simulink model "MCU_ExternalModeDataLog_dsPIC33AK128MC106"  (R2024a)
settings: Solver=FixedStepDiscrete  StartTime=0.0  StopTime=inf  FixedStep=50e-6  RelTol=1e-3  EnableMultiTasking=on
undefined symbols (not defined in the file or in its folder): A0, A4, ADC, B0, C10, C11, C6, C7, C8, control, D11, D12, DiscIntNeverNeededParam, inverter, Max, MaxPer, motor, ms, NumBits1, NumBits2, P1, P17, P20, P39, P40, P41, P43, P44, P60, P61, Pin, PosRange1, PosRange2, PWM1_Trg1, Resol, s, Slope1, Slope2, us
libraries: simulink x34, MCHP_Blockset x18
(part 1 of 5)
settings Model: SimulationMode=external  ExtModeEnableFloating=off  ExtModeTrigDuration=20  Creator=rdelpoux  LastModifiedBy=rdelpoux
settings SolverCC: AlgebraicLoopSolver=TrustRegion
settings OptimizationCC: DefaultParameterBehavior=Inlined  DefaultUnderspecifiedDataType=single  EnhancedBackFolding=on  BooleansAsBitfields=on  PassReuseOutputArgsAs=Individual arguments  ZeroExternalMemoryAtStartup=off  ZeroInternalMemoryAtStartup=off  OptimizeBlockOrder=speed  DifferentSizesBufferReuse=on  EfficientTunableParamExpr=on
settings DebuggingCC: MultiTaskDSMMsg=none  MultiTaskCondExecSysMsg=none  MultiTaskRateTransMsg=warning  ParameterTunabilityLossMsg=error  ArithmeticOperatorsInVariantConditions=warning
settings HardwareCC: ProdBitPerPointer=32  ProdBitPerSizeT=32  ProdBitPerPtrDiffT=32  ProdLargestAtomicInteger=Long  ProdWordSize=32  ProdLongLongMode=on  ProdHWDeviceType=Generic->Custom
settings ModelReferenceCC: ModelReferenceNumInstancesAllowed=Single
settings SFSimCC: MATLABDynamicMemAlloc=off  CustomCodeUndefinedFunction=UseInterfaceOnly
settings RTWCC: Description=Microchip Embedded Target dsPIC33A (real-time)  SystemTargetFile=MCHP_dsPIC33A_stf.tlc  TLCOptions=-aExtModeXCPClassicInterface=0  TemplateMakefile=MCHP_dsPIC33A.tmf  GPUComputeCapability=3.5
settings CodeAppCC: ForceParamTrailComments=on  IgnoreCustomStorageClasses=off  MaxIdLength=255  OperatorAnnotations=on  SimulinkDataObjDesc=on  SFDataObjDesc=on  InsertBlockDesc=on
settings STFCustomTargetCC: TargetLibSuffix=_lib.a  MultiwordLength=256  CombineOutputUpdateFcns=on  CombineSignalStateStructs=on  ERTCustomFileBanners=on  SupportContinuousTime=off  RemoveResetFunc=on  MATLABClassNameForMDSCustomization=Simulink.SoftwareTarget.ERTCustomization  GRTInterface=off  UseToolchainInfoCompliant=off  SystemTargetFile=MCHP_dsPIC33A_stf.tlc
settings ERTTargetCC: TargetLibSuffix=_lib.a  TargetLangStandard=C99 (ISO)  ParMdlRefBuildCompliant=off  CompOptLevelCompliant=off  ConcurrentExecutionCompliant=off  CombineSignalStateStructs=on  SupportNonInlinedSFcns=on  ModelStepFunctionPrototypeControlCompliant=off  CPPClassGenCompliant=off  UseToolchainInfoCompliant=off  ExtMode=on  ExtModeTransport=1  ExtModeStaticAlloc=on  ExtModeStaticAllocSize=2048  ExtModeMexFile=ext_xcp  ExtModeMexArgs=1 '/dev/ttyACM1' 460800 './MCU_LuenbergerObserver_dsPIC33AK128MC106.X/MCU_LuenbergerObserver_dsPIC33AK128MC106.elf'  ExtModeIntrfLevel=Level2 - Open  InlinedParameterPlacement=NonHierarchical  ERTSrcFileBannerTemplate=MCHP_dsPIC_code_template.cgt  ERTHdrFileBannerTemplate=MCHP_dsPIC_code_template.cgt  ERTDataSrcFileTemplate=MCHP_dsPIC_code_template.cgt  ERTDataHdrFileTemplate=MCHP_dsPIC_code_template.cgt  ERTCustomFileTemplate=MCHP_main.tlc  MaxLineWidth=110

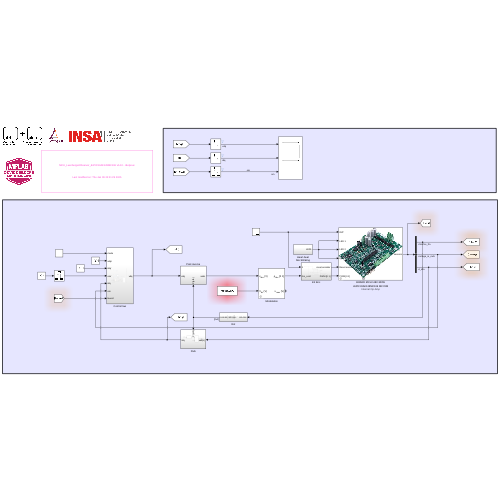
[thumbnail: Simulink's stored preview of the top-level diagram]
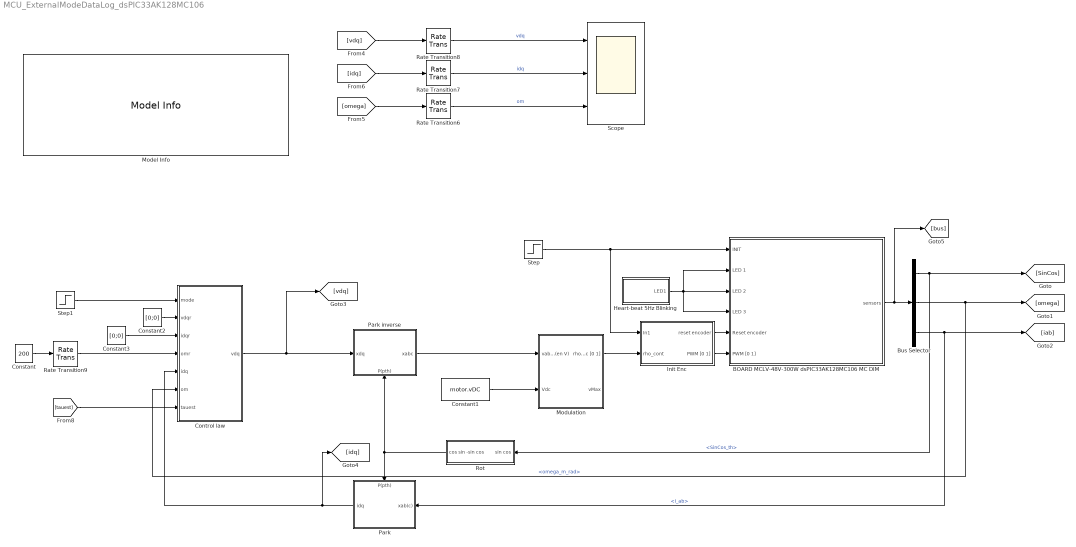
== system MCU_ExternalModeDataLog_dsPIC33AK128MC106 ==
  BOARD MCLV-48V-300W dsPIC33AK128MC106 MC DIM : Subsystem  mask(MCLV-48V-300W - dsPIC33AK128MC106 MC DIM){boardVariants=Internal Op-Amp, n=4, QEIResolution=4000, Switching_Frequency=20000, DeadTime=1e-6, QEI_Reset=on index signal, QEI_Offset_settings=0, QEIOffset=0.1885}
      mask prompts: boardVariants "Board Variants"; n "Motor Pole Pairs"; QEIResolution "Optical Encoder Resolution Per Mechanical Rotation (lines)"; Switching_Frequency "PWM Switching Frequency (Hz)"; DeadTime "Dead Time (s)"; QEI_Reset "Optical encoder reset"; QEI_Offset_settings "Optical encoder offset (mechanical in rad)"; QEIOffset "Optical encoder offset (mechanical in rad)"
      mask help:
      | Template for motor control board MCLV-48V-300W with the dsPIC33AK128MC106 Motor Control DIM.
      |
      | Block bus output provices:
      |   - Current phase ia & ib, DC bus and potentiometer position
      |   - Buttons (0 when pressed, 1 for Btn 3 unconnected)
      |   - QEI position and velocity
      |   - MCU load and overload
      |
      | Block inputs:
      |   - INIT signal average the current phase ia and ib to be removed
      |   - LEDs
      |   - Reset encoder allows to align the motor while reseting the encoder
      |   - PWM normalized duty cycle value
      |
      | Model 50us base rate (20kHz) is synchronized with ADC conversion which is synchronized with the 50us PWM periods
      mask init:
      | BlksQEI = find_system(gcb,'FollowLinks','on','LookUnderMasks','all','ReferenceBlock','MCHP_Blockset/QEI/QEI');
      | QEI_Reset = get_param(gcb,'QEI_Reset');
      | if numel(BlksQEI) >= 1
      |     switch QEI_Reset
      |         case 'on index signal'
      |             set_param(BlksQEI{1},'PIMOD_mode','RESET position on each INDEX event');
      |         case 'on logical input (software)'        
      |             set_param(BlksQEI{1},'PIMOD_mode','position is cyclique between user defined boundaries'); 
      |         case 'custom setting'
      |             % do nothing 
      |     end
      | end % if
      | 
      |     BlksOpAmp = find_system(gcb,'FollowLinks','on','IncludeCommented','on','LookUnderMasks','all','ReferenceBlock','MCHP_Blockset/Analog IO/Op-Amp');
      |     if numel(BlksOpAmp) >= 1
      |         boardVariants = get_param(gcb,'boardVariants');
      |         switch boardVariants
      |             case 'Internal Op-Amp'
      |                 set_param(BlksOpAmp{1},'Commented','off');
      |             case 'External Op-Amp'
      |                 set_param(BlksOpAmp{1},'Commented','on');
      |         end
      |     end % if
      settings: AttributesFormatString=%<boardVariants>
      mask Help: https://forum.microchip.com/s/sub-forums?&subForumId=a553l000000J2rNAAS&forumId=a553l000000J2pvAAC&subForumName=MATLAB&forumName=Development%20Tools&page=1&offset=0
      mask TypeOptions boardVariants: Internal Op-Amp | External Op-Amp
      mask TypeOptions QEI_Reset: on index signal | on logical input (software) | custom setting
      mask Callback QEI_Reset:
      | QEI_Reset = get_param(gcb,'QEI_Reset');
      | switch QEI_Reset
      |     case 'on index signal'
      |         QEIOffset = MCHP_Fun.Evalin('base','QEIOffset');
      |         set_param(gcb,'QEIOffset',num2str(QEIOffset));
      |         set_param(gcb,'MaskVisibilities',{'on';'on';'on';'on';'on';'on';'off';'on'});
      |     case 'on logical input (software)'
      |         set_param(gcb,'QEIOffset','0');
      |         set_param(gcb,'MaskVisibilities',{'on';'on';'on';'on';'on';'on';'off';'off'});
      |     case 'custom setting'
      |         set_param(gcb,'MaskVisibilities',{'on';'on';'on';'on';'on';'on';'off';'on'});
      |         % do nothing
      | end
      mask DialogControl boardParameters Prompt: Board
      mask DialogControl MotorParameters Prompt: Motor
      mask DialogControl n Tooltip: Number of pole pairs of the motor
      mask DialogControl QEIResolution Tooltip: encoder resolution per mechanical rotation
      mask DialogControl PWMParameters Prompt: PWM
      mask DialogControl QEIParameters Prompt: QEI
      mask DialogControl QEI_Reset Tooltip: enable encoder index signal if available. Otherwise align motor by applying a tension and set the rst input to 1
      mask DialogControl QEI_Offset_settings Tooltip: offset angle between encoder index and motor winding reference axis applied on theta_m and theta_e
      mask Display: image('MCHP_i_Board_MCLV_300W48V_reduced.jpg');
  Bus Selector : BusSelector  OutputSignals=optical coder.elec.SinCos_th,optical coder.mecc.omega_m_rad,ADC.I_ab
  Constant : Constant  Value=200
  Constant1 : Constant  Value=motor.vDC  OutDataTypeStr=single
  Constant2 : Constant  Value=[0;0]  OutDataTypeStr=single
  Constant3 : Constant  Value=[0;0]  OutDataTypeStr=single
  Control law : Subsystem
      settings: LibrarySourceBlock=insa_control_base/Control law
  Heart-beat 5Hz Blinking : Subsystem
  Init Enc : Subsystem
  Model Info : simulink/Model-Wide Utilities/Model Info  Frame=on  DisplayStringWithTags=|  HorizontalTextAlignment=Center  LeftAlignmentValue=0.5
      | %<ModelName> v%<ModelVersion> - %<Creator>
      | 
      | %<Description>
      | 
      | Last modified on: %<LastModificationDate>
  Modulation : Subsystem  mask{modulation=Space Vector, mod=0}
      mask init:
      | switch modulation
      |     case 'Sinusoidale'
      |         mod = 0;
      |     otherwise
      |         mod = 1;
      | end
      mask TypeOptions modulation: Sinusoidale | Space Vector
      mask DialogControl DescGroupVar Prompt: Modulation interssecticve
      mask DialogControl DescTextVar Prompt: Choose between sinus or space vector modulation
      mask Display:
      | port_label('output', 1, '\rho_{abc} [0 1]', 'texmode','on')
      | port_label('output', 2, 'v_{\rm max} (V)', 'texmode','on')
      | port_label('input', 1, 'v_{abc} (V)', 'texmode','on')
      | port_label('input', 2, 'V_{dc} (V)', 'texmode','on')
  Park : Subsystem
      settings: PortSchema="{\"entries\":[{\"content\":{\"sides\":[{\"content\":{\"connectorIds\":[\"In1\"]},\"type\":\"ConnectorPlacement.EquallySpacedRectSide\",\"uuid\":\"ebf2fcb8-f94c-4630-a735-fb74e68b604e\"},{\"content\":{\"connectorIds\":[\"Out1\"],\"side\":\"RIGHT\"},\"type\":\"ConnectorPlacement.EquallySpacedRectSide\",\"uuid\":\"fb89ad3f-9420-4065-992c-c6d77ce245e0\"},{\"content\":{\"connectorIds\":[\"In2\"],\"side\":\"TOP\"},\"type\":\"ConnectorPlacement.EquallySpacedRectSide\",\"uuid\":\"0249ceba-2241-48c9-87d4-d9d6f381f2d7\"}]},\"type\":\"ConnectorPlacement.EquallySpacedConnector\",\"uuid\":\"eecfd82d-5918-403e-a677-09fe1d8cc737\"}],\"packageUris\":[\"http://schema.mathworks.com/mf0/Connector/R2020b\"],\"version\":\"1.0\"}"
  Park inverse : Subsystem
      settings: PortSchema="{\"entries\":[{\"content\":{\"sides\":[{\"content\":{\"connectorIds\":[\"In1\"]},\"type\":\"ConnectorPlacement.EquallySpacedRectSide\",\"uuid\":\"4c11ef0a-1978-4a73-9b5c-4d5650fcee33\"},{\"content\":{\"connectorIds\":[\"Out1\"],\"side\":\"RIGHT\"},\"type\":\"ConnectorPlacement.EquallySpacedRectSide\",\"uuid\":\"28284572-70c7-45ef-9db5-4b5788e96454\"},{\"content\":{\"side\":\"TOP\"},\"type\":\"ConnectorPlacement.EquallySpacedRectSide\",\"uuid\":\"3a1fbce2-0868-491b-8e3a-2b3a7a0d615d\"},{\"content\":{\"connectorIds\":[\"In2\"],\"side\":\"BOTTOM\"},\"type\":\"ConnectorPlacement.EquallySpacedRectSide\",\"uuid\":\"e63426ef-821a-4774-a922-a3f70d9b2116\"}]},\"type\":\"ConnectorPlacement.EquallySpacedConnector\",\"uuid\":\"285593a5-8af6-47f2-83d9-d6ebce98de71\"}],\"packageUris\":[\"http://schema.mathworks.com/mf0/Connector/R2020b\"],\"version\":\"1.0\"}"
  Rate Transition6 : RateTransition  OutPortSampleTime=0.001
  Rate Transition7 : RateTransition  OutPortSampleTime=0.001
  Rate Transition8 : RateTransition  OutPortSampleTime=0.001
  Rate Transition9 : RateTransition  OutPortSampleTime=5e-5
  Rot : Subsystem
  Scope : Scope  NumInputPorts=3
  Step : Step  Before=1  After=0  SampleTime=5e-5
  Step1 : Step  After=3  SampleTime=5e-5
  wires:
  Bus Selector/2 -> [omega], Control law/6(om)  "<omega_m_rad>"
  BOARD MCLV-48V-300W dsPIC33AK128MC106 MC DIM/1(sensors) -> [bus], Bus Selector/1
  Bus Selector/1 -> Rot/1(sin cos), [SinCos]  "<SinCos_th>"
  Bus Selector/3 -> [iab], Park/1(xab(c))  "<I_ab>"
  Rot/1("cos sin -sin cos ") -> Park/2(P(pth)), Park inverse/2(P(pth))
  Constant1/1 -> Modulation/2(Vdc)
  Heart-beat 5Hz Blinking/1(LED1) -> BOARD MCLV-48V-300W dsPIC33AK128MC106 MC DIM/4(LED 3), BOARD MCLV-48V-300W dsPIC33AK128MC106 MC DIM/2(LED 1), BOARD MCLV-48V-300W dsPIC33AK128MC106 MC DIM/3(LED 2)
  Park inverse/1(xabc) -> Modulation/1("vabc (en V) ")
  Control law/1(vdq) -> Park inverse/1(xdq), [vdq]
  Park/1(idq) -> Control law/5(idq), [idq]
  [omega] -> Rate Transition6/1
  [vdq] -> Rate Transition8/1
  [idq] -> Rate Transition7/1
  Step/1 -> Init Enc/1(In1), BOARD MCLV-48V-300W dsPIC33AK128MC106 MC DIM/1(INIT)
  Constant2/1 -> Control law/2(vdqr)
  Constant3/1 -> Control law/3(idqr)
  Constant/1 -> Rate Transition9/1
  Rate Transition9/1 -> Control law/4(omr)
  Step1/1 -> Control law/1(mode)
  Modulation/1(rho_abc [0 1]) -> Init Enc/2(rho_cont)
  Init Enc/1(reset encoder) -> BOARD MCLV-48V-300W dsPIC33AK128MC106 MC DIM/5(Reset encoder)
  Init Enc/2(PWM [0 1]) -> BOARD MCLV-48V-300W dsPIC33AK128MC106 MC DIM/6(PWM [0 1])
  Rate Transition6/1 -> Scope/3  "om"
  Rate Transition8/1 -> Scope/1  "vdq"
  Rate Transition7/1 -> Scope/2  "idq"
  [tauest] -> Control law/7(tauest)
